simulink model "uro_sim"  (R2022b)
settings: Solver=FixedStepAuto  StartTime=0  StopTime=T_TO  FixedStep=Ts  RelTol=1e-3
values from neighbouring files (symbols this model uses):
  I = 3.78223425915421    (= 3.78223425915)    [real_piv_uro_exp.m]
  K_aw = 2.7    [real_piv_uro_exp.m]
  P = 0.99212598425196863    (= 0.992125984252)    [real_piv_uro_exp.m]
  Ts = 0.01    [real_piv_uro_exp.m]
  u_max = 100    [real_piv_uro_exp.m]
  u_min = -100    [real_piv_uro_exp.m]
  V = 0.83758762153302224    (= 0.837587621533)    [real_piv_uro_exp.m]
libraries: cstblocks x6
settings Model: Creator=ladislav  LastModifiedBy=ladislav

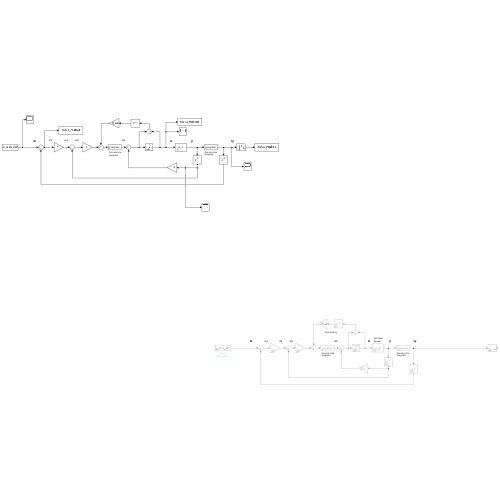
[thumbnail: Simulink's stored preview of the top-level diagram]
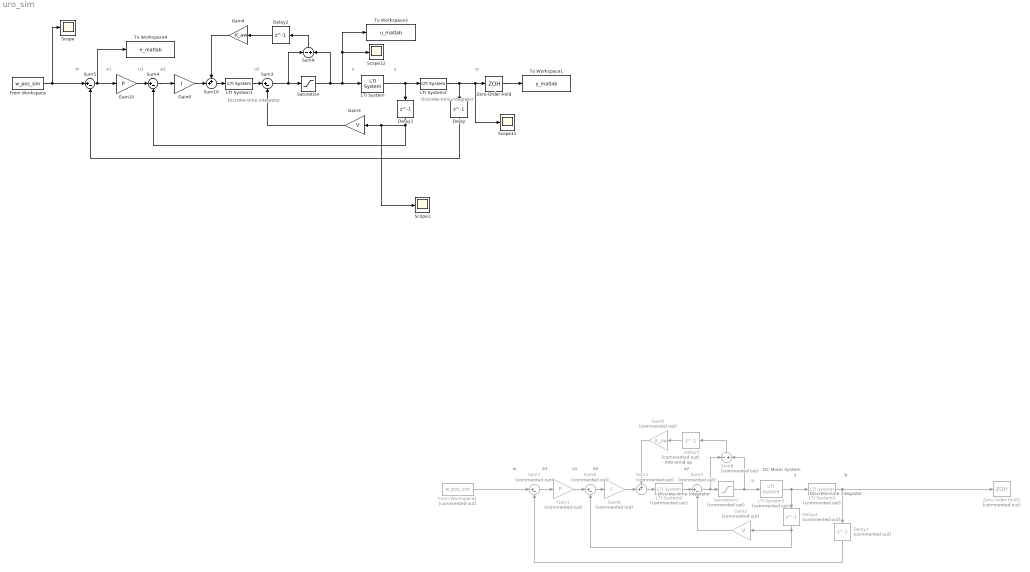
== system uro_sim ==
  note: w
  note: iy
  note: u
  note: u2
  note: e1
  note: e2
  note: u1
  note: y
  note: Discrete-time integrator
  note: Discrete-time integrator
  note: Discrete-time integrator
  note: iy
  note: Discrete-time integrator
  note: y
  note: e1
  note: u2
  note: u
  note: e2
  note: u1
  note: w
  note: DC Motor
      | System
  note: Anti-wind up
  Delay : Delay  DelayLength=1
  Delay1 : Delay  DelayLength=1
  Delay2 : Delay  DelayLength=1
  Delay3 : Delay  Commented=on  DelayLength=1
  Delay4 : Delay  Commented=on  DelayLength=1
  Delay5 : Delay  Commented=on  DelayLength=1
  From Workspace : FromWorkspace  VariableName=w_pos_sim  SampleTime=Ts
  From Workspace1 : FromWorkspace  Commented=on  VariableName=w_pos_sim  SampleTime=Ts
  Gain1 : Gain  Commented=on  Gain=P
  Gain10 : Gain  Gain=P
  Gain2 : Gain  Commented=on  Gain=V
  Gain3 : Gain  Gain=V
  Gain4 : Gain  Gain=K_aw
  Gain5 : Gain  Commented=on  Gain=K_aw
  Gain6 : Gain  Commented=on  Gain=I
  Gain9 : Gain  Gain=I
  LTI System : cstblocks/LTI System  sys=G_Z  IC=[]
  LTI System1 : cstblocks/LTI System  sys=Integrator  IC=[]
  LTI System2 : cstblocks/LTI System  sys=Integrator  IC=[]
  LTI System3 : cstblocks/LTI System  Commented=on  sys=G_Z  IC=[]
  LTI System4 : cstblocks/LTI System  Commented=on  sys=Integrator  IC=[]
  LTI System5 : cstblocks/LTI System  Commented=on  sys=Integrator  IC=[]
  Saturation : Saturate  UpperLimit=u_max  LowerLimit=u_min  LinearizeAsGain=off
  Saturation1 : Saturate  Commented=on  UpperLimit=u_max  LowerLimit=u_min  LinearizeAsGain=off
  Scope{,1,11..12} (4 alike) : Scope
  Sum1 : Sum  Commented=on  Inputs=++|
  Sum10 : Sum  Inputs=++|
  Sum2 : Sum  Commented=on  Inputs=|+-
  Sum3 : Sum  Inputs=|+-
  Sum4 : Sum  Inputs=|+-
  Sum5 : Sum  Inputs=|+-
  Sum6 : Sum  Commented=on  Inputs=|+-
  Sum7 : Sum  Commented=on  Inputs=|+-
  Sum8 : Sum  Commented=on  Inputs=-|+
  Sum9 : Sum  Inputs=-|+
  To Workspace1 : ToWorkspace  VariableName=y_matlab  SaveFormat=Timeseries  SampleTime=-1
  To Workspace3 : ToWorkspace  VariableName=u_matlab  SaveFormat=Timeseries  SampleTime=-1
  To Workspace4 : ToWorkspace  VariableName=e_matlab  SaveFormat=Timeseries  SampleTime=-1
  Zero-Order Hold : ZeroOrderHold  SampleTime=0.01
  Zero-Order Hold1 : ZeroOrderHold  Commented=on  SampleTime=0.01
  wires:
  Sum5/1 -> To Workspace4/1, Gain10/1
  Gain3/1 -> Sum3/2
  LTI System/1 -> Delay1/1, LTI System2/1
  LTI System1/1 -> Sum3/1
  Sum3/1 -> Sum9/1, Saturation/1
  Gain10/1 -> Sum4/1
  From Workspace/1 -> Sum5/1, Scope/1
  LTI System2/1 -> Scope11/1, Zero-Order Hold/1, Delay/1
  Sum4/1 -> Gain9/1
  Sum10/1 -> LTI System1/1
  Gain9/1 -> Sum10/2
  Sum9/1 -> Delay2/1
  Delay/1 -> Sum5/2
  Delay1/1 -> Scope1/1, Gain3/1, Sum4/2
  Gain4/1 -> Sum10/1
  Delay2/1 -> Gain4/1
  Saturation/1 -> Sum9/2, Scope12/1, To Workspace3/1, LTI System/1
  Zero-Order Hold/1 -> To Workspace1/1
  Sum2/1 -> Saturation1/1, Sum8/1
  LTI System3/1 -> LTI System5/1, Delay4/1
  Delay5/1 -> Gain5/1
  Delay4/1 -> Gain2/1, Sum6/2
  Saturation1/1 -> LTI System3/1, Sum8/2
  Sum6/1 -> Gain6/1
  Gain6/1 -> Sum1/2
  From Workspace1/1 -> Sum7/1
  Gain5/1 -> Sum1/1
  LTI System4/1 -> Sum2/1
  Sum1/1 -> LTI System4/1
  LTI System5/1 -> Zero-Order Hold1/1, Delay3/1
  Gain2/1 -> Sum2/2
  Gain1/1 -> Sum6/1
  Sum7/1 -> Gain1/1
  Delay3/1 -> Sum7/2
  Sum8/1 -> Delay5/1
